simulink model "DCMotor"  (R2023a)
settings: Solver=VariableStepAuto  StartTime=0.0  StopTime=10.0  RelTol=1e-3
InitFcn:
  | Lab2Rob
values from neighbouring files (symbols this model uses):
  Km = .191    (= 0.191)    [InitialCons.m]
  La = 2.5e-3    (= 0.0025)    [InitialCons.m]
  Ra = 14.69    [InitialCons.m]
  tm = 0.0095    [InitialCons.m]    (also in torque.m)
settings Model: Creator=willi  LastModifiedBy=willi

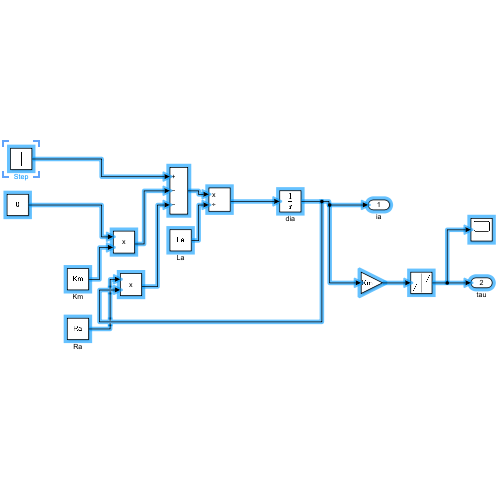
[thumbnail: Simulink's stored preview of the top-level diagram]
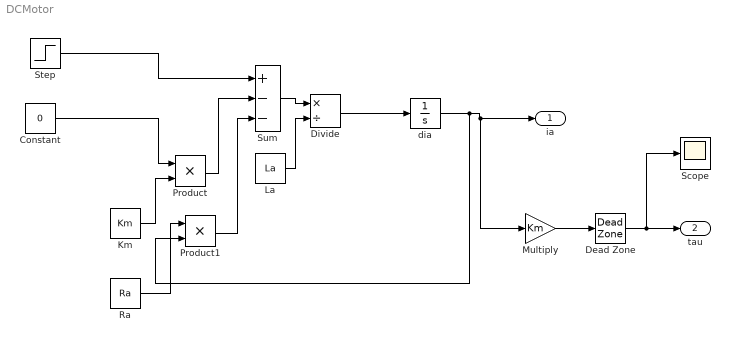
== system DCMotor ==
  Constant : Constant  Value=0
  Dead Zone : DeadZone  LowerValue=-tm  UpperValue=tm
  Divide : Product  Inputs=*/
  Km : Constant  Value=Km
  La : Constant  Value=La
  Multiply : Gain  Gain=Km
  Product : Product
  Product1 : Product
  Ra : Constant  Value=Ra
  Scope : Scope
  Step : Step  After=12  SampleTime=0
  Sum : Sum  Inputs=+--
  dia : Integrator
  ia : Outport
  tau : Outport  Port=2
  wires:
  dia/1 -> Multiply/1, ia/1, Product1/2
  Step/1 -> Sum/1
  Constant/1 -> Product/1
  Km/1 -> Product/2
  Sum/1 -> Divide/1
  Ra/1 -> Product1/1
  Product1/1 -> Sum/3
  Divide/1 -> dia/1
  Product/1 -> Sum/2
  La/1 -> Divide/2
  Multiply/1 -> Dead Zone/1
  Dead Zone/1 -> Scope/1, tau/1
